simulink model "invarianza_temporal"  (R2020b)
settings: Solver=VariableStepAuto  StartTime=0.0  StopTime=8  MaxStep=1e-2  RelTol=1e-3
settings Model: Creator=carma  LastModifiedBy=carma
settings DataIOCC: ReturnWorkspaceOutputs=off
settings DebuggingCC: ArithmeticOperatorsInVariantConditions=warning
settings SFSimCC: SimUseLocalCustomCode=off  CustomCodeUndefinedFunction=UseInterfaceOnly
settings RTWCC: RTWUseLocalCustomCode=off

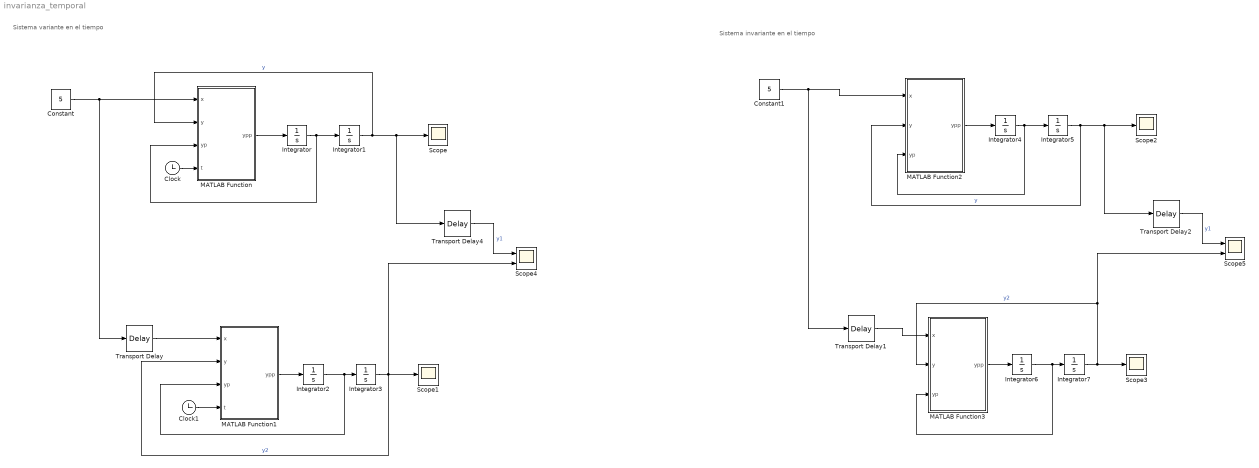
== system invarianza_temporal ==
  note: Sistema variante en el tiempo
  note: Sistema invariante en el tiempo
  Clock : Clock
  Clock1 : Clock
  Constant : Constant  Value=5
  Constant1 : Constant  Value=5
  Integrator{,1..7} (8 alike) : Integrator
  MATLAB Function : MATLAB Function  TreatAsAtomicUnit=on
  MATLAB Function1 : MATLAB Function  TreatAsAtomicUnit=on
  MATLAB Function2 : MATLAB Function  TreatAsAtomicUnit=on
  MATLAB Function3 : MATLAB Function  TreatAsAtomicUnit=on
  Scope{,1..3} (4 alike) : Scope
  Scope4 : Scope  NumInputPorts=2
  Scope5 : Scope  NumInputPorts=2
  Transport Delay{,1..2,4} (4 alike) : TransportDelay
  wires:
  MATLAB Function/1(ypp) -> Integrator/1
  Integrator/1 -> Integrator1/1, MATLAB Function/3(yp)
  Integrator1/1 -> MATLAB Function/2(y), Transport Delay4/1, Scope/1  "y"
  Clock/1 -> MATLAB Function/4(t)
  Constant/1 -> Transport Delay/1, MATLAB Function/1(x)
  Integrator3/1 -> Scope4/2, MATLAB Function1/2(y), Scope1/1  "y2"
  Clock1/1 -> MATLAB Function1/4(t)
  Integrator2/1 -> MATLAB Function1/3(yp), Integrator3/1
  MATLAB Function1/1(ypp) -> Integrator2/1
  Transport Delay4/1 -> Scope4/1  "y1"
  Transport Delay/1 -> MATLAB Function1/1(x)
  MATLAB Function3/1(ypp) -> Integrator6/1
  Transport Delay1/1 -> MATLAB Function3/1(x)
  Integrator7/1 -> Scope5/2, MATLAB Function3/2(y), Scope3/1  "y2"
  Transport Delay2/1 -> Scope5/1  "y1"
  Constant1/1 -> Transport Delay1/1, MATLAB Function2/1(x)
  Integrator6/1 -> MATLAB Function3/3(yp), Integrator7/1
  Integrator4/1 -> Integrator5/1, MATLAB Function2/3(yp)
  Integrator5/1 -> MATLAB Function2/2(y), Transport Delay2/1, Scope2/1  "y"
  MATLAB Function2/1(ypp) -> Integrator4/1

== matlab function invarianza_temporal/MATLAB Function1 ==
  data: x input; ypp output; y input; yp input; t input
function ypp = fcn(x,y,yp,t)

ypp =2*x-8*y-4*t*yp;

== matlab function invarianza_temporal/MATLAB Function ==
  data: x input; ypp output; y input; yp input; t input
function ypp = fcn(x,y,yp,t)

ypp =2*x-8*y-4*t*yp;

== matlab function invarianza_temporal/MATLAB Function2 ==
  data: x input; ypp output; y input; yp input
function ypp = fcn(x,y,yp)

ypp =2*x-8*y-4*yp;

== matlab function invarianza_temporal/MATLAB Function3 ==
  data: x input; ypp output; y input; yp input
function ypp = fcn(x,y,yp)

ypp =2*x-8*y-4*yp;
